simulink model "working_kalman"  (R2025b)
settings: Solver=FixedStepDiscrete  StartTime=0.0  StopTime=+inf  FixedStep=simulink_Ts  RelTol=1e-3  EnableMultiTasking=on
InitFcn:
  | InitSensorFusion
values from neighbouring files (symbols this model uses):
  acc_calib_matrix = [0.9990,0.0039,0.0028;4.2507e-04,0.9990,-0.0085;0.0015,0.0090,0.9997]    [InitSensorFusion.m]
  avg_order = 2    [InitSensorFusion.m]
  calibration_time = 10    [InitSensorFusion.m]
  d = 0.15*sqrt(2)/2    [InitSensorFusion.m]
  friction_offset = 0.0001    [InitSensorFusion.m]
  friction_slope = 20e-6    (= 2e-05)    [InitSensorFusion.m]
  g = 9.81    [InitSensorFusion.m]
  ground_true_g = 9.81275    [InitSensorFusion.m]
  Ic0 = Is0 + Iw0 - Iwg    [InitSensorFusion.m]
  ICM42_gyr_offset = [-0.1319, -0.6878, 0.1737]    [InitSensorFusion.m]
  ICM42_params = SUPER_PARAMS    [InitSensorFusion.m]
  init_acc_bias = [-0.0076;0.0233;0.0477]    [InitSensorFusion.m]
  init_P = P_initial    [InitSensorFusion.m]
  init_rot_quat = [0 0 0 1]'    [InitSensorFusion.m]
  Iwg = 315e-6    (= 0.000315)    [InitSensorFusion.m]
  kalman_Ts = 0.01    [InitSensorFusion.m]
  KV = 330    [InitSensorFusion.m]
  mc = mw + ms    (= 0.75)    [InitSensorFusion.m]
  sensor_Ts = 0.01    [InitSensorFusion.m]
  simulink_Ts = 0.01    [InitSensorFusion.m]
  stateInit = StateEnum.Initialization    [InitSensorFusion.m]
undefined symbols (not defined in the file or in its folder): acc_init_bias, init_time, StateEnum
libraries: mbedblockslib x25, simulink x12, nucleoutilitieslib x10, stmnucleof7lib x7, canmsglib x6, simulink_extras x2, visionstatistics x2
(part 1 of 2)
settings Model: SimulationMode=external  ExtModeTrigDuration=10  Creator=dozav  LastModifiedBy=dozav
settings SolverCC: AutoInsertRateTranBlk=on
settings DataIOCC: SaveOutput=off  DSMLogging=off  ReturnWorkspaceOutputs=off  LoggingFileName=loggedData.mat
settings OptimizationCC: EnhancedBackFolding=on  PassReuseOutputArgsAs=Individual arguments  ZeroExternalMemoryAtStartup=off  ZeroInternalMemoryAtStartup=off  MaxStackSize=64  OptimizeBlockOrder=speed  DifferentSizesBufferReuse=on  OptimizationCustomize=off  EfficientTunableParamExpr=on
settings DebuggingCC: ParameterTunabilityLossMsg=error
settings HardwareCC: ProdBitPerPointer=32.0  ProdBitPerSizeT=32.0  ProdBitPerPtrDiffT=32.0  ProdLargestAtomicInteger=Long  ProdLargestAtomicFloat=Double  ProdWordSize=32.0  ProdLongLongMode=on  ProdHWDeviceType=ARM Compatible->ARM Cortex-M
settings ModelReferenceCC: UpdateModelReferenceTargets=Force
settings SFSimCC: MATLABDynamicMemAlloc=off
settings RTWCC: SystemTargetFile=ert.tlc  HardwareBoard=STM32 Nucleo F767ZI  TemplateMakefile=ert_default_tmf  Toolchain=GNU Tools for ARM Embedded Processors  Description=Embedded Coder
settings CodeAppCC: ForceParamTrailComments=on  IgnoreCustomStorageClasses=off  OperatorAnnotations=on  SimulinkDataObjDesc=on  SFDataObjDesc=on  InsertBlockDesc=on
settings ERTTargetCC: ExtModeTransport=3.0  ExtModeStaticAlloc=on  ExtModeStaticAllocSize=2000.0  ExtModeMexFile=ext_xcp  ExtModeIntrfLevel=Level2 - Open  InlinedParameterPlacement=Hierarchical  TargetLangStandard=C99 (ISO)

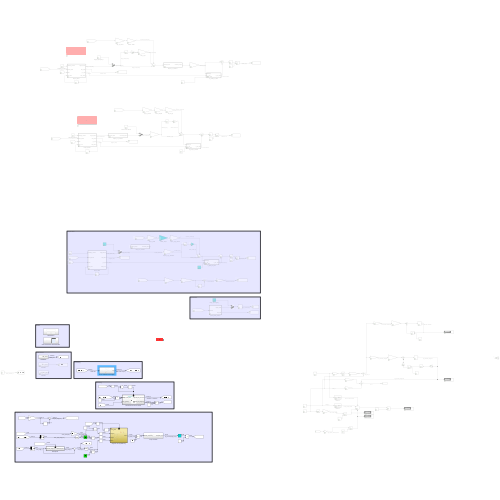
[thumbnail: Simulink's stored preview of the top-level diagram]
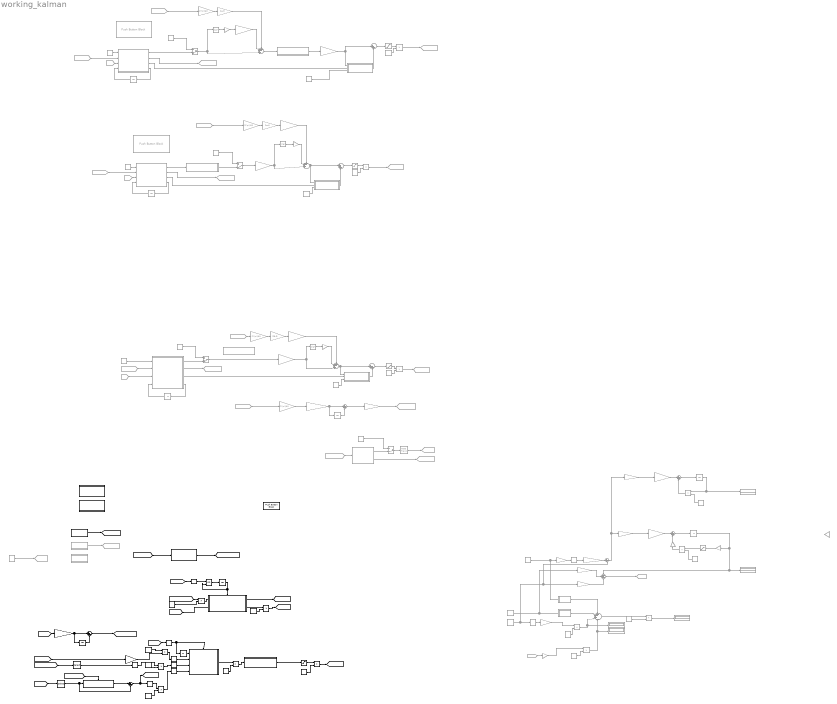
== system working_kalman ==
  note: Regulation
  note: Torque stairs
  note: Speed stairs
  note: Utilities
  note: Estimating
  note: Processing
  note: Measurement
  CAN communication with B-G431-ESC1 : Subsystem
  Constant{1,8..9,16,21} (5 alike) : Constant
  Constant{2,4,6,10..12,19..20} (8 alike) : Constant  Commented=on
  Constant13 : Constant  Commented=on  Value=0
  Constant14 : Constant  Commented=on  Value=0
  Constant15 : Constant  Commented=on  Value=0
  Constant17 : Constant  Value=-1
  Constant18 : Constant  Value=-1
  Constant3 : Constant  Commented=on  Value=5
  Constant5 : Constant  Commented=on  Value=5
  Constant7 : Constant  Commented=on  Value=5
  Degrees to Radians : simulink_extras/Transformations/Degrees to Radians
  Degrees to Radians1 : simulink_extras/Transformations/Degrees to Radians
  Display{,1..4} (5 alike) : Display  Commented=on
  Friction2 : Subsystem  Commented=on
  Friction3 : Subsystem  Commented=on
  From : From  Commented=on  GotoTag=seconds_counter  TagVisibility=global
  From{10..11,13..14,16..17,19} (7 alike) : From  Commented=on  GotoTag=wheel_speed  TagVisibility=global
  From12 : From  Commented=on  GotoTag=state  TagVisibility=global
  From15 : From  Commented=on  GotoTag=state  TagVisibility=global
  From18 : From  Commented=on  GotoTag=state  TagVisibility=global
  From29 : From  Commented=on  GotoTag=v
  Gain : Gain  Gain=1/kalman_Ts
  Gain1 : Gain  Gain=2*pi/60
  Gain10 : Gain  Commented=on  Gain=(2*pi*KV)/60
  Gain11 : Gain  Commented=on  Gain=0.2
  Gain12 : Gain  Commented=on  Gain=11
  Gain13 : Gain  Commented=on  Gain=Ic0
  Gain14 : Gain  Commented=on  Gain=Ic0
  Gain15 : Gain  Commented=on  Gain=-36
  Gain16 : Gain  Commented=on  Gain=-0.02
  Gain17 : Gain  Commented=on  Gain=1/Ic0
  Gain18 : Gain  Commented=on  Gain=Ic0
  Gain19 : Gain  Commented=on  Gain=mc*g*d
  Gain2 : Gain  Commented=on  Gain=simulink_Ts
  Gain20 : Gain  Commented=on  Gain=0.15
  Gain22 : Gain  Commented=on  Gain=-36
  Gain24 : Gain  Commented=on  Gain=simulink_Ts
  Gain3 : Gain  Commented=on  Gain=1/(simulink_Ts*2)
  Gain4 : Gain  Commented=on  Gain=36
  Gain5 : Gain  Commented=on  Gain=Iwg
  Gain6 : Gain  Commented=on  Gain=(2*pi)/60
  Gain7 : Gain  Commented=on  Gain=0.2
  Gain8 : Gain  Commented=on  Gain=(2*pi*KV)/60
  Gain9 : Gain  Commented=on  Gain=0.2
  Goto10 : Goto  Commented=on  GotoTag=applied_torque
  Goto{7,11..12,14} (4 alike) : Goto  Commented=on  GotoTag=program_stop  TagVisibility=global
  Goto13 : Goto  Commented=on  GotoTag=ramp_torque  TagVisibility=global
  Goto15 : Goto  Commented=on  GotoTag=ramp_torque  TagVisibility=global
  Goto16 : Goto  Commented=on  GotoTag=check_timer
  Goto17 : Goto  Commented=on  GotoTag=v
  Goto5 : Goto  Commented=on  GotoTag=MPU_AccGyr
  Goto6 : Goto  Commented=on  GotoTag=ramp_speed  TagVisibility=global
  Goto9 : Goto  Commented=on  GotoTag=ramp_torque  TagVisibility=global
  ICM20948 : Subsystem  Commented=on
  ICM42688-P : Subsystem
  Iq_peak_for_start : MATLAB Function  Commented=on  TreatAsAtomicUnit=on
  Iq_peak_for_start1 : MATLAB Function  Commented=on  TreatAsAtomicUnit=on
  Iq_peak_for_start2 : MATLAB Function  Commented=on  TreatAsAtomicUnit=on
  Kalman Sensor Fusion for ICM42 : Subsystem
  MPU6050 : Subsystem  Commented=on
  Manual Switch{,1..3} (4 alike) : ManualSwitch  Commented=on  CurrentSetting=0
  New Setpoint : Subsystem
  Nm_to_Iq1 : Gain  Commented=on  Gain=1/((2*pi*KV)/60)
  Nm_to_Iq2 : Gain  Commented=on  Gain=(2*pi*KV)/60
  OR : Logic  Operator=OR  IconShape=distinctive  AllPortsSameDT=off  OutDataTypeStr=boolean
  Product{,4..5,10..12,14} (7 alike) : Product
  Product{1..3,6..9,13} (8 alike) : Product  Commented=on
  Push Button : PushButtonBlock  ButtonText=Start/Stop  IconOnColor=[0.0, 0.39215686274509803, 0.0]  IconOffColor=[0.0, 1.0, 0.0]  OffValue=0.000000
  Push Button1 : PushButtonBlock  Commented=on  ButtonText=Start/Stop  IconOnColor=[0.0, 0.39215686274509803, 0.0]  IconOffColor=[0.0, 1.0, 0.0]  OffValue=0.000000
  Push Button2 : PushButtonBlock  Commented=on  ButtonText=Start/Stop  IconOnColor=[0.0, 0.39215686274509803, 0.0]  IconOffColor=[0.0, 1.0, 0.0]  OffValue=0.000000
  Rate Transition{,1..3} (4 alike) : RateTransition  OutPortSampleTime=simulink_Ts
  Rate Transition4 : RateTransition  Commented=on  OutPortSampleTime=simulink_Ts
  Rate Transition5 : RateTransition  OutPortSampleTime=kalman_Ts
  Regulation for Edge Balancing : Subsystem
  Saturation : Saturate  UpperLimit=4  LowerLimit=-4
  Saturation1 : Saturate  Commented=on  UpperLimit=4.5  LowerLimit=-4.5
  Saturation2 : Saturate  Commented=on  UpperLimit=1.8  LowerLimit=-1.8
  Saturation3 : Saturate  Commented=on  UpperLimit=1.8  LowerLimit=-1.8
  Saturation4 : Saturate  Commented=on
  Selector : Selector  InputPortWidth=3  IndexOptions=Index vector (dialog)  Indices=[3]  OutputSizes=1
  Selector1 : Selector  InputPortWidth=3  IndexOptions=Index vector (dialog)  Indices=[3]  OutputSizes=1
  Sensor Calibration and Averaging : Subsystem
  Sign : Signum  Commented=on
  Sign1 : Signum  Commented=on
  Sign2 : Signum  Commented=on
  Sin3 : Trigonometry  Commented=on
  State Machine : Subsystem
  Sum : Sum  Inputs=|+-
  Sum1 : Sum  Inputs=|+-
  Sum10 : Sum  Commented=on  Inputs=---
  Sum11 : Sum  Commented=on  Inputs=|+-
  Sum12 : Sum  Commented=on  Inputs=+|-|+|-
  Sum{4,6,8..9,13} (5 alike) : Sum  Commented=on  Inputs=|++
  Sum2 : Sum  Commented=on  Inputs=|+-
  Sum3 : Sum  Commented=on  Inputs=+++|
  Sum5 : Sum  Commented=on  Inputs=+++|
  Sum7 : Sum  Commented=on  Inputs=+++|
  Tanh1 : Trigonometry  Commented=on  Operator=tanh
  Torque Correction : Subsystem
  Unit Delay : UnitDelay  SampleTime=-1  HasFrameUpgradeWarning=on
  Unit Delay{1..2,6..8} (5 alike) : UnitDelay  Commented=on  SampleTime=simulink_Ts  HasFrameUpgradeWarning=on
  Unit Delay3 : UnitDelay  InitialCondition=zeros(1,3)  SampleTime=kalman_Ts  HasFrameUpgradeWarning=on
  Unit Delay4 : UnitDelay  SampleTime=simulink_Ts  HasFrameUpgradeWarning=on
  Unit Delay5 : UnitDelay  Commented=on  SampleTime=simulink_Ts*2  HasFrameUpgradeWarning=on
  friction_slope : Gain  Commented=on  Gain=2e-5
  friction_slope1 : Gain  Commented=on  Gain=2e-5
  friction_slope2 : Gain  Commented=on  Gain=2e-5
  manual_target_torque [Nm] : Constant  Commented=on  Value=0.01  OutDataTypeStr=single
  rpm_to_rad/s : Gain  Commented=on  Gain=(2*pi)/60
  rpm_to_rad/s1 : Gain  Commented=on  Gain=(2*pi)/60
  rpm_to_rad/s2 : Gain  Commented=on  Gain=(2*pi)/60
  sampling_counter{,1..3} (4 alike) : simulink/Sources/Counter Free-Running  Commented=on  NumBits=32  tsamp=simulink_Ts
  speed_stairs_function : MATLAB Function  Commented=on  TreatAsAtomicUnit=on
  target_speed [rpm] : Constant  Commented=on  Value=1500  OutDataTypeStr=single
  target_torque [Nm]1 : Constant  Commented=on  Value=0.01  OutDataTypeStr=single
  target_torque [Nm]2 : Constant  Commented=on  Value=0.01  OutDataTypeStr=single
  torque_inv_function : MATLAB Function  Commented=on  TreatAsAtomicUnit=on
  torque_inv_function1 : MATLAB Function  Commented=on  TreatAsAtomicUnit=on
  torque_inv_function2 : MATLAB Function  Commented=on  TreatAsAtomicUnit=on
  torque_stairs : MATLAB Function  Commented=on  TreatAsAtomicUnit=on
  torque_stairs1 : MATLAB Function  Commented=on  TreatAsAtomicUnit=on
  torque_stairs2 : MATLAB Function  Commented=on  TreatAsAtomicUnit=on
  torque_to_Iq_corrected : Gain  Commented=on  Gain=(2*pi*KV)/60
  torque_to_Iq_friction : Gain  Commented=on  Gain=(2*pi*KV)/60
  tag scope: ICM42_EA=global, ICM42_rot_q=global, error_angle=global, ramp_torque=global
  wires:
  ICM42688-P/1(ICM_AccGyr) -> [ICM42_AccGyr]  "ICM42_data"
  [ICM42_g] -> Kalman Sensor Fusion for ICM42/2(used_g [m/s^2])
  MPU6050/1(MPU_AccGyr) -> Goto5/1
  [isIdle] -> Rate Transition5/1
  OR/1 -> Unit Delay/1
  [ICM42_AccGyr] -> Sensor Calibration and Averaging/1(In1)  "ICM42_data"
  Sensor Calibration and Averaging/1(avg) -> [ICM42_AccGyr_avg]  "ICM42_data_avg"
  Kalman Sensor Fusion for ICM42/1(Out1) -> [ICM42_rot_q]  "estimated_rot_quaternion"
  Gain/1 -> Sum/1, Unit Delay3/1
  [wheel_speed] -> Gain1/1  "wheel_speed [rpm]"
  Sum/1 -> [ICM42_EA_omega]  "ICM_EA_omega [°/s]"
  Torque Correction/1(corrected_Iq [A]) -> Saturation/1  "reg_corrected_target_Iq [A]"
  [ICM42_EA] -> Gain/1
  [ICM42_EA_omega] -> Selector1/1
  Selector1/1 -> Degrees to Radians/1  "euler_angle_omega [°/s]"
  Unit Delay3/1 -> Sum/2
  Sum1/1 -> [error_angle], Degrees to Radians1/1  "error_angle [°]"
  Product/1 -> [ramp_torque]
  Constant1/1 -> Product/2
  Rate Transition/1 -> Regulation for Edge Balancing/4(theta c)
  Rate Transition1/1 -> Regulation for Edge Balancing/3(omega c)
  [isRunning] -> Rate Transition3/1
  Rate Transition3/1 -> Regulation for Edge Balancing/Enable, Unit Delay4/1
  Unit Delay4/1 -> Regulation for Edge Balancing/1(running_label)
  From/1 -> speed_stairs_function/1(seconds)
  speed_stairs_function/2(stop_start) -> Goto7/1
  speed_stairs_function/1(target_speed) -> Manual Switch/2
  Manual Switch/1 -> Rate Transition4/1
  target_speed [rpm]/1 -> Manual Switch/1
  Rate Transition4/1 -> Goto6/1  "target_speed [rpm]"
  manual_target_torque [Nm]/1 -> Manual Switch1/1
  Gain3/1 -> Sum2/1, Unit Delay5/1
  Unit Delay5/1 -> Sum2/2
  Gain6/1 -> Gain3/1
  Sum2/1 -> Gain5/1  "rot_accel [rad/s^2]"
  Gain5/1 -> Goto10/1  "applied_torque [Nm]"
  From10/1 -> Gain6/1
  torque_stairs/2(stop_start) -> Goto11/1  "program_stop"
  torque_stairs/1(target_torque) -> Manual Switch1/2  "target_torque [Nm]"
  Saturation1/1 -> Product1/1
  Constant2/1 -> Product1/2
  Product1/1 -> Goto9/1  "target_Iq [A]"
  Manual Switch1/1 -> torque_to_Iq_corrected/1  "target_torque [Nm]"
  sampling_counter/1 -> torque_stairs/1(sampling_counter)
  From11/1 -> torque_stairs/2(wheel_speed)
  From12/1 -> torque_stairs/3(state)
  torque_stairs/4(step_done) -> Unit Delay6/1
  Unit Delay6/1 -> torque_stairs/4("step_done ")
  torque_stairs/3(t_in_slot) -> Iq_peak_for_start/2(t_in_slot)  "t_in_slot [s]"
  torque_to_Iq_corrected/1 -> Sum3/3, Sign/1  "desired_Iq [A]"
  Constant3/1 -> Iq_peak_for_start/3(decay_slope)
  Sign/1 -> Gain7/1
  Sum3/1 -> Iq_peak_for_start/1(desired_Iq), Sum4/1
  Iq_peak_for_start/1(Iq_for_start) -> Sum4/2  "Iq_peak_ampl [A]"
  Sum4/1 -> Saturation1/1
  From13/1 -> rpm_to_rad/s/1
  Gain7/1 -> Sum3/2  "static_friction [A]"
  rpm_to_rad/s/1 -> friction_slope/1
  friction_slope/1 -> torque_to_Iq_friction/1
  torque_to_Iq_friction/1 -> Sum3/1  "dynamic_friction [A]"
  friction_slope1/1 -> Sum5/1  "dynamic_torque [Nm]"
  Product2/1 -> Goto13/1  "target_Iq [A]"
  Sum5/1 -> torque_inv_function1/1(desired_torque)
  torque_stairs1/2(stop_start) -> Goto12/1  "program_stop"
  target_torque [Nm]1/1 -> Manual Switch2/1
  Sign1/1 -> Gain9/1
  torque_stairs1/1(target_torque) -> Manual Switch2/2  "target_torque [Nm]"
  From14/1 -> torque_stairs1/2(wheel_speed)
  Manual Switch2/1 -> Sum5/3, Sign1/1  "target_torque [Nm]"
  Saturation2/1 -> Product2/1
  Constant4/1 -> Product2/2
  From15/1 -> torque_stairs1/3(state)
  Constant5/1 -> Iq_peak_for_start1/3(decay_slope)
  Unit Delay7/1 -> torque_stairs1/4("step_done ")
  rpm_to_rad/s1/1 -> friction_slope1/1
  Sum6/1 -> Saturation2/1
  torque_stairs1/3(t_in_slot) -> Iq_peak_for_start1/2(t_in_slot)  "t_in_slot [s]"
  Iq_peak_for_start1/1(Iq_for_start) -> Sum6/2  "Iq_peak_ampl [A]"
  sampling_counter1/1 -> torque_stairs1/1(sampling_counter)
  From16/1 -> rpm_to_rad/s1/1
  Gain9/1 -> Nm_to_Iq1/1  "static_friction [A]"
  torque_stairs1/4(step_done) -> Unit Delay7/1
  Nm_to_Iq1/1 -> Sum5/2  "static_torque [Nm]"
  Gain8/1 -> Sum6/1, Iq_peak_for_start1/1(desired_Iq)  "desired_Iq [A]"
  torque_inv_function1/1(corrected_torque) -> Gain8/1
  friction_slope2/1 -> Nm_to_Iq2/1
  Gain10/1 -> Sign2/1, Sum7/3  "desired_Iq [A]"
  Unit Delay8/1 -> torque_stairs2/4("step_done ")
  Sum7/1 -> Iq_peak_for_start2/1(desired_Iq), Sum8/1
  torque_stairs2/2(stop_start) -> Goto14/1  "program_stop"
  torque_stairs2/3(t_in_slot) -> Iq_peak_for_start2/2(t_in_slot)  "t_in_slot [s]"
  From18/1 -> torque_stairs2/3(state)
  Constant7/1 -> Iq_peak_for_start2/3(decay_slope)
  Gain11/1 -> Sum7/2  "static_friction [A]"
  From17/1 -> torque_stairs2/2(wheel_speed)
  Constant6/1 -> Product3/2
  target_torque [Nm]2/1 -> Manual Switch3/1
  rpm_to_rad/s2/1 -> friction_slope2/1
  Sum8/1 -> Saturation3/1
  From19/1 -> rpm_to_rad/s2/1
  torque_stairs2/4(step_done) -> Unit Delay8/1
  Nm_to_Iq2/1 -> Sum7/1  "dynamic_friction [A]"
  sampling_counter2/1 -> torque_stairs2/1(sampling_counter)
  Product3/1 -> Goto15/1  "target_Iq [A]"
  Sign2/1 -> Gain11/1
  Saturation3/1 -> Product3/1
  torque_inv_function2/1(corrected_torque) -> Manual Switch3/2
  torque_stairs2/1(target_torque) -> torque_inv_function2/1(desired_torque)  "target_torque [Nm]"
  Manual Switch3/1 -> Gain10/1  "target_torque [Nm]"
  Iq_peak_for_start2/1(Iq_for_start) -> Sum8/2  "Iq_peak_ampl [A]"
  Saturation/1 -> Product/1
  sampling_counter3/1 -> Goto16/1  "timer_simulink_Ts"
  Constant8/1 -> Product4/2
  Regulation for Edge Balancing/1(torque) -> Product4/1  "reg_target_torque [Nm]"
  Product4/1 -> Torque Correction/1(desired_torque [Nm])
  Constant9/1 -> Product5/2
  Kalman Sensor Fusion for ICM42/2(EA) -> Product5/1  "estimated_euler_angles [°]"
  Product5/1 -> [ICM42_EA]
  Rate Transition2/1 -> Regulation for Edge Balancing/2(omega w)
  Constant16/1 -> Product10/1
  Gain1/1 -> Product10/2  "wheel_speed [rad/s]"
  Product10/1 -> Rate Transition2/1
  Sum9/1 -> Unit Delay1/1
  Sin3/1 -> Gain19/1
  Product7/1 -> Display/1
  Gain20/1 -> Tanh1/1
  Gain2/1 -> Sum9/1
  Sum10/1 -> Goto17/1  "reg_v"
  Gain16/1 -> Sum11/1
  Tanh1/1 -> Gain16/1
  Gain12/1 -> Sum10/2
  Gain18/1 -> Product8/1  "reg_torque_fictional_action"
  Constant19/1 -> Product6/2
  Sum12/1 -> Product7/1
  Constant12/1 -> Product9/2
  Constant11/1 -> Product7/2
  Gain19/1 -> Product9/1  "reg_torque_gravity"
  Constant15/1 -> Gain12/1, Friction3/1(rad/s)  "omega_c"
  Unit Delay1/1 -> Display4/1, Sum10/1, Gain13/1  "reg_discrete_integrator"
  Constant13/1 -> Friction2/1(rad/s), Gain20/1
  Friction3/1(friction) -> Sum12/2  "torque_cubli_friction"
  Constant14/1 -> Gain4/1, Sum11/2, Sin3/1  "theta_c"
  From29/1 -> Gain18/1
  Gain4/1 -> Sum10/3
  Product6/1 -> Gain17/1
  Product9/1 -> Sum12/3, Display1/1
  Product8/1 -> Display2/1, Sum12/4
  Constant10/1 -> Product8/2
  Friction2/1(friction) -> Sum12/1  "torque_wheel_friction"
  Constant17/1 -> Product11/2
  Degrees to Radians1/1 -> Product11/1  "error_euler_angle [rad]"
  Product11/1 -> Rate Transition/1
  Constant18/1 -> Product12/2
  Degrees to Radians/1 -> Product12/1  "euler_angle_omega [rad/s]"
  Product12/1 -> Rate Transition1/1
  Saturation4/1 -> Product6/1
  Sum11/1 -> Gain22/1, Gain15/1  "reg_thc_err"
  Gain15/1 -> Gain2/1  "reg_discrete_integrator"
  Gain13/1 -> Saturation4/1
  Gain17/1 -> Sum9/2
  Constant20/1 -> Product13/2
  Gain22/1 -> Gain24/1  "reg_discrete_integrator"
  Gain24/1 -> Sum13/1
  Sum13/1 -> Unit Delay2/1
  Unit Delay2/1 -> Display3/1, Product13/1  "reg_discrete_integrator"
  Product13/1 -> Sum13/2
  Constant21/1 -> Product14/2
  [ICM42_AccGyr_avg] -> Product14/1
  Product14/1 -> Kalman Sensor Fusion for ICM42/1(meased_data_6axis)
  Unit Delay/1 -> OR/2, Kalman Sensor Fusion for ICM42/Enable
  Rate Transition5/1 -> OR/1
  [isSettingSetpoint] -> New Setpoint/Enable
  [ICM42_EA] -> Selector/1
  Selector/1 -> New Setpoint/1(measured_angle [°]), Sum1/2  "euler_angle [°]"
  New Setpoint/1(setpoint_angle [°]) -> Sum1/1  "target_angle [°]"

== system working_kalman/CAN communication with B-G431-ESC1 ==
  Receive CAN Messages : Subsystem
  Send CAN Messages : Subsystem

== system working_kalman/Friction2 ==
  rad/s : Inport
  Gain : Gain  Gain=300
  Gain1 : Gain  Gain=friction_offset
  Gain2 : Gain  Gain=friction_slope
  Gain4 : Gain  Gain=1/(2*pi*60)
  Sum : Sum  Inputs=|++
  Tanh : Trigonometry  Operator=tanh
  friction : Outport
  wires:
  rad/s/1 -> Gain4/1
  Gain4/1 -> Gain2/1, Gain/1  "rpm"
  Gain1/1 -> Sum/1
  Tanh/1 -> Gain1/1
  Gain2/1 -> Sum/2
  Gain/1 -> Tanh/1
  Sum/1 -> friction/1

== system working_kalman/Friction3 ==
  rad/s : Inport
  Gain : Gain  Gain=300
  Gain1 : Gain  Gain=friction_offset
  Gain2 : Gain  Gain=friction_slope
  Gain4 : Gain  Gain=1/(2*pi*60)
  Sum : Sum  Inputs=|++
  Tanh : Trigonometry  Operator=tanh
  friction : Outport
  wires:
  rad/s/1 -> Gain4/1
  Gain4/1 -> Gain2/1, Gain/1  "rpm"
  Gain1/1 -> Sum/1
  Tanh/1 -> Gain1/1
  Gain2/1 -> Sum/2
  Gain/1 -> Tanh/1
  Sum/1 -> friction/1

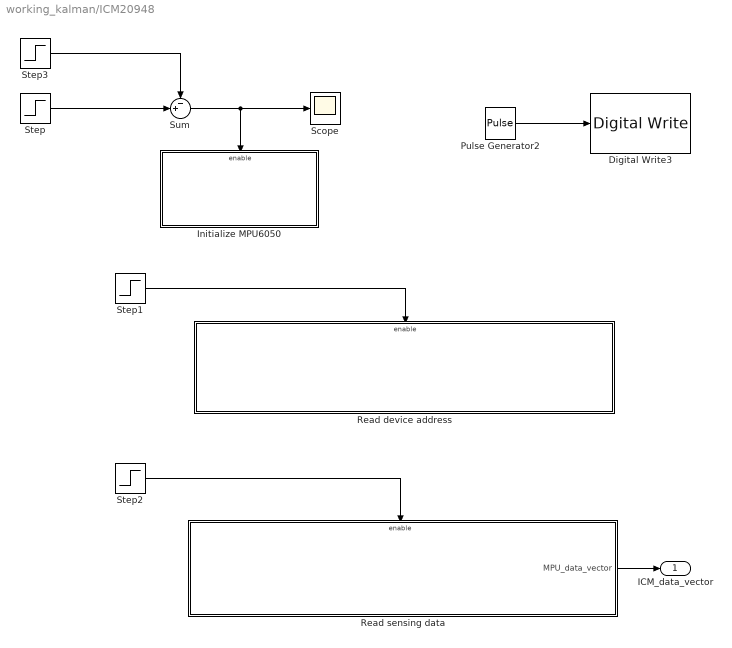
== system working_kalman/ICM20948 ==
  Digital Write3 : mbedblockslib/Digital Write  Pin=LED3  Direction=output
      settings: LibrarySourceBlock=stmnucleorootlib/Common/Digital Write
  Initialize MPU6050 : Subsystem
  Pulse Generator2 : DiscretePulseGenerator  PulseType=Time based  PulseWidth=50
  Read device address : Subsystem
  Read sensing data : Subsystem
  Scope : Scope
      settings: DataLoggingVariableName=ScopeData5
  Step : Step
  Step1 : Step  Time=2
  Step2 : Step  Time=2
  Step3 : Step  Time=1.5
  Sum : Sum  Inputs=-+|
  ICM_data_vector : Outport
  wires:
  Step2/1 -> Read sensing data/Enable
  Read sensing data/1(MPU_data_vector) -> ICM_data_vector/1
  Sum/1 -> Scope/1, Initialize MPU6050/Enable
  Step/1 -> Sum/2
  Step1/1 -> Read device address/Enable
  Step3/1 -> Sum/1
  Pulse Generator2/1 -> Digital Write3/1

== system working_kalman/ICM42688-P ==
  Measurement : Subsystem
  OR : Logic  Operator=OR  IconShape=distinctive  AllPortsSameDT=off  OutDataTypeStr=boolean
  Range and sensitivity : Subsystem  Priority=1
  Selector : Selector  InputPortWidth=7  IndexOptions=Starting index (dialog)  Indices=[2]  OutputSizes=6
  Step1 : Step  Time=init_time - 3
  Step3 : Step  Time=init_time - 4
  Unit Delay : UnitDelay  SampleTime=-1  HasFrameUpgradeWarning=on
  Waking up : Subsystem  Priority=2
  ICM_AccGyr : Outport
  wires:
  Step1/1 -> Waking up/Trigger
  Step3/1 -> Range and sensitivity/Trigger
  OR/1 -> Unit Delay/1
  Unit Delay/1 -> OR/2, Measurement/Enable
  Measurement/1(ICM_data_vector) -> Selector/1
  [isCalibrating] -> OR/1
  Selector/1 -> ICM_AccGyr/1

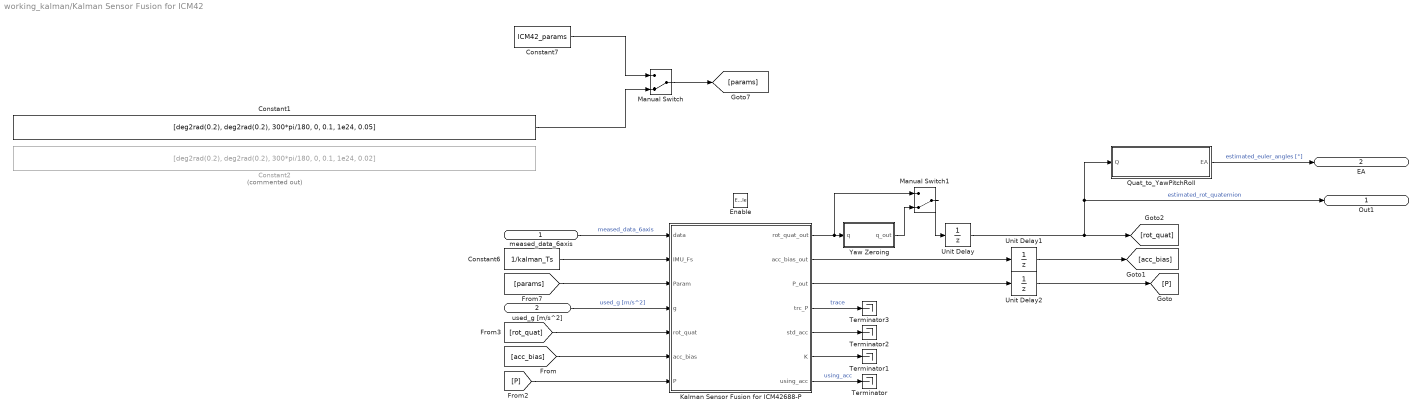
== system working_kalman/Kalman Sensor Fusion for ICM42 ==
  meased_data_6axis : Inport
  used_g [m/s^2] : Inport  Port=2
  Enable : EnablePort
  Constant1 : Constant  Value=[deg2rad(0.2), deg2rad(0.2), 300*pi/180, 0, 0.1, 1e24, 0.05]  SampleTime=-1
  Constant2 : Constant  Commented=on  Value=[deg2rad(0.2), deg2rad(0.2), 300*pi/180, 0, 0.1, 1e24, 0.02]  SampleTime=-1
  Constant6 : Constant  Value=1/kalman_Ts  SampleTime=kalman_Ts
  Constant7 : Constant  Value=ICM42_params  SampleTime=-1
  Kalman Sensor Fusion for ICM42688-P : MATLAB Function  TreatAsAtomicUnit=on  SystemSampleTime=kalman_Ts
  Manual Switch : ManualSwitch  CurrentSetting=0
  Manual Switch1 : ManualSwitch  CurrentSetting=0
  Quat_to_YawPitchRoll : MATLAB Function  TreatAsAtomicUnit=on
  Terminator{,1..3} (4 alike) : Terminator
  Unit Delay : UnitDelay  InitialCondition=init_rot_quat  SampleTime=kalman_Ts  HasFrameUpgradeWarning=on
  Unit Delay1 : UnitDelay  InitialCondition=init_acc_bias  SampleTime=kalman_Ts  HasFrameUpgradeWarning=on
  Unit Delay2 : UnitDelay  InitialCondition=init_P*eye(7)  SampleTime=kalman_Ts  HasFrameUpgradeWarning=on
  Yaw Zeroing : MATLAB Function  TreatAsAtomicUnit=on
  Out1 : Outport
  EA : Outport  Port=2
  wires:
  [acc_bias] -> Kalman Sensor Fusion for ICM42688-P/6(acc_bias)
  [P] -> Kalman Sensor Fusion for ICM42688-P/7(P)
  Unit Delay/1 -> Quat_to_YawPitchRoll/1(Q), Out1/1, [rot_quat]  "estimated_rot_quaternion"
  [rot_quat] -> Kalman Sensor Fusion for ICM42688-P/5(rot_quat)
  Kalman Sensor Fusion for ICM42688-P/2(acc_bias_out) -> Unit Delay1/1
  Kalman Sensor Fusion for ICM42688-P/3(P_out) -> Unit Delay2/1
  [params] -> Kalman Sensor Fusion for ICM42688-P/3(Param)
  Unit Delay1/1 -> [acc_bias]
  Unit Delay2/1 -> [P]
  meased_data_6axis/1 -> Kalman Sensor Fusion for ICM42688-P/1(data)  "meased_data_6axis"
  used_g [m/s^2]/1 -> Kalman Sensor Fusion for ICM42688-P/4(g)  "used_g [m/s^2]"
  Quat_to_YawPitchRoll/1(EA) -> EA/1  "estimated_euler_angles [°]"
  Constant6/1 -> Kalman Sensor Fusion for ICM42688-P/2(IMU_Fs)
  Constant7/1 -> Manual Switch/1
  Constant1/1 -> Manual Switch/2
  Manual Switch/1 -> [params]
  Kalman Sensor Fusion for ICM42688-P/7(using_acc) -> Terminator/1  "using_acc"
  Kalman Sensor Fusion for ICM42688-P/4(trc_P) -> Terminator3/1  "trace"
  Kalman Sensor Fusion for ICM42688-P/5(std_acc) -> Terminator2/1
  Kalman Sensor Fusion for ICM42688-P/6(K) -> Terminator1/1
  Kalman Sensor Fusion for ICM42688-P/1(rot_quat_out) -> Manual Switch1/1, Yaw Zeroing/1(q)
  Manual Switch1/1 -> Unit Delay/1
  Yaw Zeroing/1(q_out) -> Manual Switch1/2

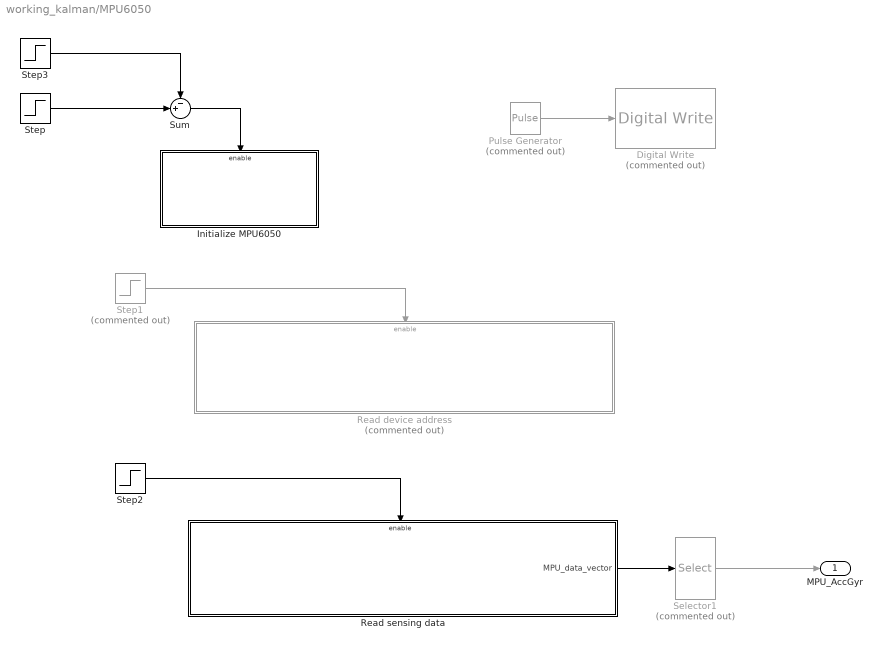
== system working_kalman/MPU6050 ==
  Digital Write : mbedblockslib/Digital Write  Commented=on  Pin=LED1  Direction=output
      settings: LibrarySourceBlock=stmnucleorootlib/Common/Digital Write
  Initialize MPU6050 : Subsystem
  Pulse Generator : DiscretePulseGenerator  Commented=on  PulseType=Time based  Period=0.5  PulseWidth=50
  Read device address : Subsystem  Commented=on
  Read sensing data : Subsystem
  Selector1 : Selector  Commented=on  InputPortWidth=7  IndexOptions=Index vector (dialog)  Indices=[1 2 3 5 6 7]  OutputSizes=6
  Step : Step
  Step1 : Step  Commented=on  Time=2
  Step2 : Step  Time=2
  Step3 : Step  Time=1.5
  Sum : Sum  Inputs=-+|
  MPU_AccGyr : Outport
  wires:
  Step2/1 -> Read sensing data/Enable
  Read sensing data/1(MPU_data_vector) -> Selector1/1
  Sum/1 -> Initialize MPU6050/Enable
  Step/1 -> Sum/2
  Pulse Generator/1 -> Digital Write/1
  Step1/1 -> Read device address/Enable
  Step3/1 -> Sum/1
  Selector1/1 -> MPU_AccGyr/1

== system working_kalman/New Setpoint ==
  measured_angle [°] : Inport
  Enable : EnablePort
  setpoint_angle [°] : Outport  InitialOutput=0
  wires:
  measured_angle [°]/1 -> setpoint_angle [°]/1

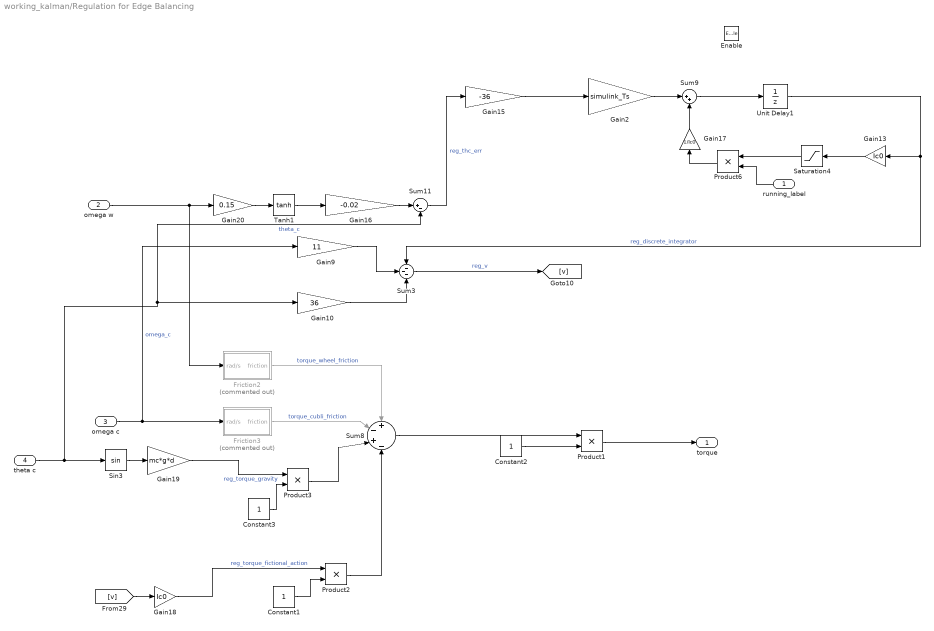
== system working_kalman/Regulation for Edge Balancing ==
  running_label : Inport
  omega w : Inport  Port=2
  omega c : Inport  Port=3
  theta c : Inport  Port=4
  Enable : EnablePort
  Constant1 : Constant
  Constant2 : Constant
  Constant3 : Constant
  Friction2 : Subsystem  Commented=on
  Friction3 : Subsystem  Commented=on
  Gain10 : Gain  Gain=36
  Gain13 : Gain  Gain=Ic0
  Gain15 : Gain  Gain=-36
  Gain16 : Gain  Gain=-0.02
  Gain17 : Gain  Gain=1/Ic0
  Gain18 : Gain  Gain=Ic0
  Gain19 : Gain  Gain=mc*g*d
  Gain2 : Gain  Gain=simulink_Ts
  Gain20 : Gain  Gain=0.15
  Gain9 : Gain  Gain=11
  Product{1..3,6} (4 alike) : Product
  Saturation4 : Saturate
  Sin3 : Trigonometry
  Sum11 : Sum  Inputs=|+-
  Sum3 : Sum  Inputs=---
  Sum8 : Sum  Inputs=+|-|+|-
  Sum9 : Sum  Inputs=|++
  Tanh1 : Trigonometry  Operator=tanh
  Unit Delay1 : UnitDelay  SampleTime=simulink_Ts  HasFrameUpgradeWarning=on
  torque : Outport
  wires:
  omega c/1 -> Gain9/1, Friction3/1(rad/s)  "omega_c"
  Sin3/1 -> Gain19/1
  Sum3/1 -> [v]  "reg_v"
  Friction2/1(friction) -> Sum8/1  "torque_wheel_friction"
  Product1/1 -> torque/1
  Gain16/1 -> Sum11/1
  Gain10/1 -> Sum3/3
  Constant2/1 -> Product1/2
  Tanh1/1 -> Gain16/1
  Friction3/1(friction) -> Sum8/2  "torque_cubli_friction"
  Gain20/1 -> Tanh1/1
  [v] -> Gain18/1
  omega w/1 -> Friction2/1(rad/s), Gain20/1
  Sum8/1 -> Product1/1
  theta c/1 -> Gain10/1, Sum11/2, Sin3/1  "theta_c"
  Gain9/1 -> Sum3/2
  Constant1/1 -> Product2/2
  Gain18/1 -> Product2/1  "reg_torque_fictional_action"
  Product2/1 -> Sum8/4
  Constant3/1 -> Product3/2
  Gain19/1 -> Product3/1  "reg_torque_gravity"
  Product3/1 -> Sum8/3
  Gain15/1 -> Gain2/1
  Gain13/1 -> Saturation4/1
  Saturation4/1 -> Product6/1
  Unit Delay1/1 -> Sum3/1, Gain13/1  "reg_discrete_integrator"
  Gain2/1 -> Sum9/1
  Sum9/1 -> Unit Delay1/1
  Product6/1 -> Gain17/1
  Gain17/1 -> Sum9/2
  running_label/1 -> Product6/2
  Sum11/1 -> Gain15/1  "reg_thc_err"

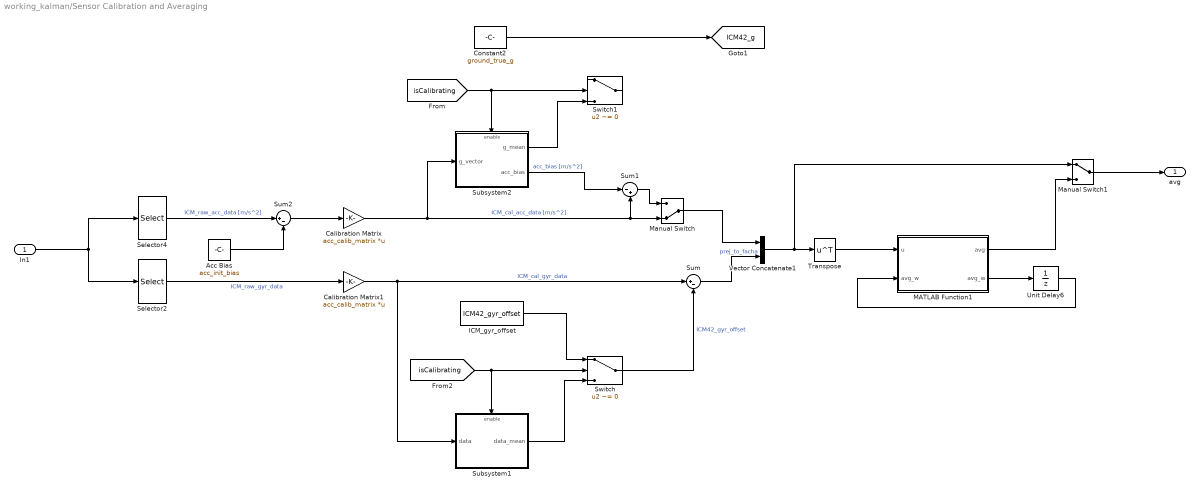
== system working_kalman/Sensor Calibration and Averaging ==
  In1 : Inport
  Acc Bias : Constant  Value=acc_init_bias  SampleTime=simulink_Ts
  Calibration Matrix : Gain  Gain=acc_calib_matrix  Multiplication=Matrix(K*u)
  Calibration Matrix1 : Gain  Gain=acc_calib_matrix  Multiplication=Matrix(K*u)
  Constant2 : Constant  Value=ground_true_g  SampleTime=kalman_Ts
  ICM_gyr_offset : Constant  Value=ICM42_gyr_offset  SampleTime=-1
  MATLAB Function1 : MATLAB Function  TreatAsAtomicUnit=on
  Manual Switch : ManualSwitch  CurrentSetting=0
  Manual Switch1 : ManualSwitch
  Selector2 : Selector  InputPortWidth=6  IndexOptions=Starting index (dialog)  Indices=[4]  OutputSizes=3
  Selector4 : Selector  InputPortWidth=6  IndexOptions=Starting index (dialog)  Indices=[1]  OutputSizes=3
  Subsystem1 : Subsystem
  Subsystem2 : Subsystem
  Sum : Sum  Inputs=|+-
  Sum1 : Sum  Inputs=|-+
  Sum2 : Sum  Inputs=|+-
  Switch : Switch  Criteria=u2 ~= 0  Threshold=111  SaturateOnIntegerOverflow=off  InputSameDT=off
  Switch1 : Switch  Criteria=u2 ~= 0  SaturateOnIntegerOverflow=off  InputSameDT=off
  Transpose : Math  Operator=transpose
  Unit Delay6 : UnitDelay  InitialCondition=zeros(avg_order, 6)  SampleTime=-1  HasFrameUpgradeWarning=on
  Vector Concatenate1 : Concatenate
  avg : Outport
  tag scope: ICM42_g=global
  wires:
  Subsystem1/1(data_mean) -> Switch/3
  In1/1 -> Selector2/1, Selector4/1
  MATLAB Function1/2(avg_w) -> Unit Delay6/1
  Vector Concatenate1/1 -> Manual Switch1/1, Transpose/1
  Selector2/1 -> Calibration Matrix1/1  "ICM_raw_gyr_data"
  [isCalibrating] -> Subsystem2/Enable, Switch1/2
  Subsystem2/1(g_mean) -> Switch1/3
  Unit Delay6/1 -> MATLAB Function1/2("avg_w ")
  ICM_gyr_offset/1 -> Switch/1
  [isCalibrating] -> Switch/2, Subsystem1/Enable
  Switch/1 -> Sum/2  "ICM42_gyr_offset"
  Sum/1 -> Vector Concatenate1/2  "prej_to_facha"
  Transpose/1 -> MATLAB Function1/1(u)
  Subsystem2/2(acc_bias) -> Sum1/1  "acc_bias [m/s^2]"
  Manual Switch/1 -> Vector Concatenate1/1
  Sum1/1 -> Manual Switch/1
  Calibration Matrix/1 -> Sum1/2, Manual Switch/2, Subsystem2/1(g_vector)  "ICM_cal_acc_data [m/s^2]"
  Selector4/1 -> Sum2/1  "ICM_raw_acc_data [m/s^2]"
  Sum2/1 -> Calibration Matrix/1
  Acc Bias/1 -> Sum2/2
  Constant2/1 -> [ICM42_g]
  Calibration Matrix1/1 -> Sum/1, Subsystem1/1(data)  "ICM_cal_gyr_data"
  MATLAB Function1/1(avg) -> Manual Switch1/2
  Manual Switch1/1 -> avg/1

== system working_kalman/State Machine ==
  State Recognition : Subsystem
  State Signalizition : Subsystem
  State Updates : Subsystem

== system working_kalman/Torque Correction ==
  desired_torque [Nm] : Inport
  Gain12 : Gain  Gain=(2*pi*KV)/60
  Gain13 : Gain  Gain=0.2
  Sign3 : Signum
  Sum9 : Sum  Inputs=+++|
  friction_slope3 : Gain  Gain=2e-5
  friction_torque_to_Iq1 : Gain  Gain=(2*pi*KV)/60
  rpm_to_rad/s3 : Gain  Gain=(2*pi)/60
  torque_inv_function3 : MATLAB Function  TreatAsAtomicUnit=on
  corrected_Iq [A] : Outport
  wires:
  Gain13/1 -> Sum9/2  "offset_for_dynamic_friction [A]"
  rpm_to_rad/s3/1 -> friction_slope3/1
  torque_inv_function3/1(corrected_torque) -> Gain12/1  "corrected_torque [Nm]"
  [wheel_speed] -> rpm_to_rad/s3/1
  Gain12/1 -> Sum9/3, Sign3/1  "desired_Iq [A]"
  Sign3/1 -> Gain13/1
  friction_torque_to_Iq1/1 -> Sum9/1  "dynamic_friction [A]"
  friction_slope3/1 -> friction_torque_to_Iq1/1
  desired_torque [Nm]/1 -> torque_inv_function3/1(desired_torque)  "desired_torque [Nm]"
  Sum9/1 -> corrected_Iq [A]/1  "corrected_Iq [A]"

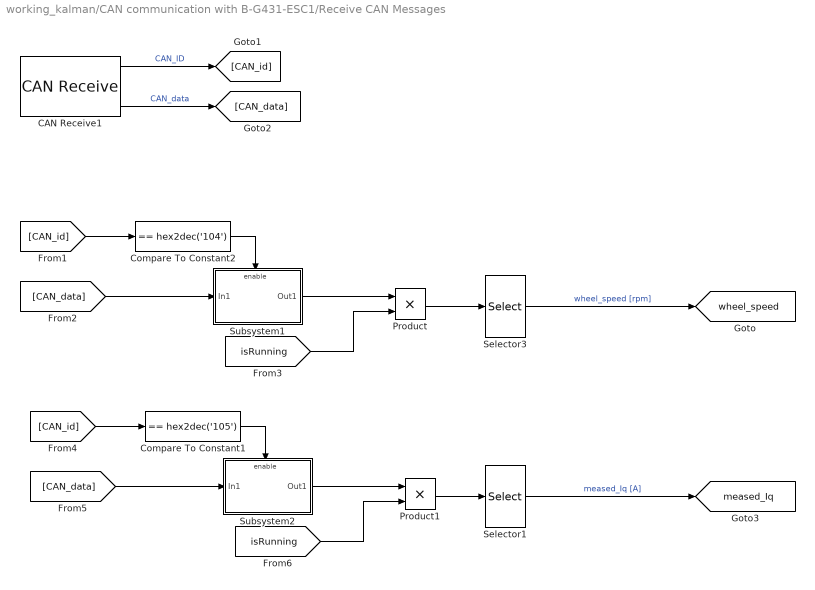
== system working_kalman/CAN communication with B-G431-ESC1/Receive CAN Messages ==
  CAN Receive1 : stmnucleof7lib/CAN Receive  CANModule=1  OutputType=Unpacked  ReadSource=FIFO 0  SampleTime=simulink_Ts  OutputIdType=off  RemoteFrame=off  OutputStatus=off
  Compare To Constant1 : simulink/Logic and Bit Operations/Compare To Constant  relop===  const=hex2dec('105')  OutDataTypeStr=boolean
  Compare To Constant2 : simulink/Logic and Bit Operations/Compare To Constant  relop===  const=hex2dec('104')  OutDataTypeStr=boolean
  Product : Product
  Product1 : Product
  Selector1 : Selector  InputPortWidth=2  IndexOptions=Starting index (dialog)  Indices=[1]  OutputSizes=1
  Selector3 : Selector  InputPortWidth=2  IndexOptions=Starting index (dialog)  Indices=[1]  OutputSizes=1
  Subsystem1 : Subsystem
  Subsystem2 : Subsystem
  tag scope: meased_Iq=global, wheel_speed=global
  wires:
  CAN Receive1/3 -> [CAN_data]  "CAN_data"
  Compare To Constant2/1 -> Subsystem1/Enable
  [CAN_id] -> Compare To Constant2/1
  [CAN_data] -> Subsystem1/1(In1)
  CAN Receive1/1 -> [CAN_id]  "CAN_ID"
  Subsystem1/1(Out1) -> Product/1
  Product/1 -> Selector3/1
  [isRunning] -> Product/2
  [isRunning] -> Product1/2
  Subsystem2/1(Out1) -> Product1/1
  Product1/1 -> Selector1/1
  Compare To Constant1/1 -> Subsystem2/Enable
  [CAN_data] -> Subsystem2/1(In1)
  [CAN_id] -> Compare To Constant1/1
  Selector3/1 -> [wheel_speed]  "wheel_speed [rpm]"
  Selector1/1 -> [meased_Iq]  "meased_Iq [A]"

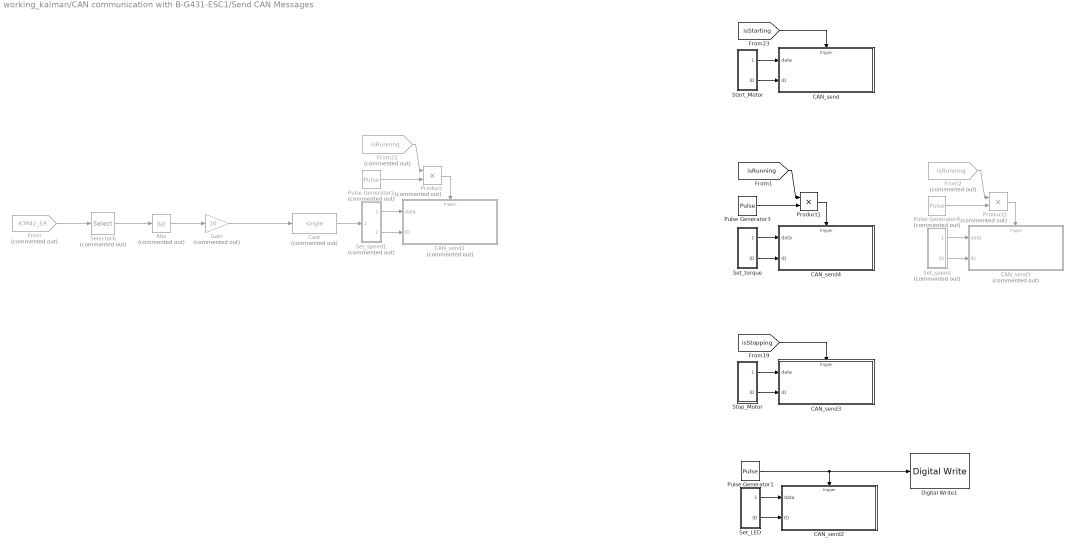
== system working_kalman/CAN communication with B-G431-ESC1/Send CAN Messages ==
  Abs : Abs  Commented=on  SaturateOnIntegerOverflow=off
  CAN_send : Subsystem
  CAN_send1 : Subsystem  Commented=on
  CAN_send2 : Subsystem
  CAN_send3 : Subsystem
  CAN_send4 : Subsystem
  CAN_send5 : Subsystem  Commented=on
  Cast : DataTypeConversion  Commented=on  OutDataTypeStr=single  SaturateOnIntegerOverflow=off  RndMeth=Floor
  Digital Write1 : mbedblockslib/Digital Write  Pin=LED1  Direction=output
      settings: LibrarySourceBlock=stmnucleorootlib/Common/Digital Write
  From : From  Commented=on  GotoTag=ICM42_EA  TagVisibility=global
  From2 : From  Commented=on  GotoTag=isRunning  TagVisibility=global
  From22 : From  Commented=on  GotoTag=isRunning  TagVisibility=global
  Gain : Gain  Commented=on  Gain=10
  Product : Product  Commented=on
  Product1 : Product
  Product2 : Product  Commented=on
  Pulse Generator1 : DiscretePulseGenerator  PulseType=Time based  Period=0.1  PulseWidth=50
  Pulse Generator2 : DiscretePulseGenerator  Commented=on  PulseType=Time based  Period=0.1  PulseWidth=50
  Pulse Generator3 : DiscretePulseGenerator  PulseType=Time based  Period=2*simulink_Ts  PulseWidth=50
  Pulse Generator4 : DiscretePulseGenerator  Commented=on  PulseType=Time based  Period=2*simulink_Ts  PulseWidth=50
  Selector6 : Selector  Commented=on  InputPortWidth=3  IndexOptions=Index vector (dialog)  Indices=[1]  OutputSizes=1
  Set_LED : Subsystem
  Set_speed : Subsystem  Commented=on
  Set_speed1 : Subsystem  Commented=on
  Set_torque : Subsystem
  Start_Motor : Subsystem
  Stop_Motor : Subsystem
  wires:
  Set_speed1/2(ID) -> CAN_send1/2(ID)
  Selector6/1 -> Abs/1
  Set_LED/1(data) -> CAN_send2/1(data)
  Stop_Motor/1(data) -> CAN_send3/1(data)
  Set_speed1/1(data) -> CAN_send1/1(data)
  [isStopping] -> CAN_send3/Trigger
  Pulse Generator1/1 -> Digital Write1/1, CAN_send2/Trigger
  Start_Motor/2(ID) -> CAN_send/2(ID)
  [isStarting] -> CAN_send/Trigger
  From22/1 -> Product/1
  Gain/1 -> Cast/1
  Start_Motor/1(data) -> CAN_send/1(data)
  Cast/1 -> Set_speed1/1(In1)
  Pulse Generator2/1 -> Product/2
  Abs/1 -> Gain/1
  Product/1 -> CAN_send1/Trigger
  Stop_Motor/2(ID) -> CAN_send3/2(ID)
  Set_LED/2(ID) -> CAN_send2/2(ID)
  From/1 -> Selector6/1
  Pulse Generator3/1 -> Product1/2
  [isRunning] -> Product1/1
  Set_torque/1(data) -> CAN_send4/1(data)
  Set_torque/2(ID) -> CAN_send4/2(ID)
  Product1/1 -> CAN_send4/Trigger
  Product2/1 -> CAN_send5/Trigger
  From2/1 -> Product2/1
  Pulse Generator4/1 -> Product2/2
  Set_speed/2(ID) -> CAN_send5/2(ID)
  Set_speed/1(data) -> CAN_send5/1(data)

== system working_kalman/ICM20948/Initialize MPU6050 ==
  Enable : EnablePort
  Accelerometer scale : mbedblockslib/I2C Controller Write  Commented=on  I2CModule=0  Mode=Master  SlaveAddress=hex2dec('68')  SlaveByteOrder=BigEndian  Direction=Transmitter  RegisterAddressMode=on  RegisterAddress=hex2dec('1C')  SlaveDataType=uint8  DataLength=2  NoAck=off  RepeatedStart=off  OutputStatus=on
      settings: LibrarySourceBlock=stmnucleorootlib/Common/I2C Controller Write
  Constant : Constant  Commented=on  Value=0b00000000
  Constant1 : Constant  Commented=on  Value=0b00001000
  Constant2 : Constant  Commented=on  Value=0b00010000
  Display1 : Display  Commented=on
  Display2 : Display  Commented=on
  Display5 : Display  Commented=on
  Gyroscope scale : mbedblockslib/I2C Controller Write  Commented=on  I2CModule=0  Mode=Master  SlaveAddress=hex2dec('68')  SlaveByteOrder=BigEndian  Direction=Transmitter  RegisterAddressMode=on  RegisterAddress=hex2dec('1B')  SlaveDataType=uint8  DataLength=2  NoAck=off  RepeatedStart=off  OutputStatus=on
      settings: LibrarySourceBlock=stmnucleorootlib/Common/I2C Controller Write
  Wake up : mbedblockslib/I2C Controller Write  Commented=on  I2CModule=0  Mode=Master  SlaveAddress=hex2dec('68')  SlaveByteOrder=BigEndian  Direction=Transmitter  RegisterAddressMode=on  RegisterAddress=hex2dec('6B')  SlaveDataType=uint8  DataLength=2  NoAck=off  RepeatedStart=off  OutputStatus=on
      settings: LibrarySourceBlock=stmnucleorootlib/Common/I2C Controller Write
  wires:
  Constant/1 -> Wake up/1
  Wake up/1 -> Display5/1
  Gyroscope scale/1 -> Display1/1
  Constant1/1 -> Gyroscope scale/1
  Constant2/1 -> Accelerometer scale/1
  Accelerometer scale/1 -> Display2/1

== system working_kalman/ICM20948/Read device address ==
  Enable : EnablePort
  Display1 : Display  Commented=on
  Display2 : Display
  Display3 : Display  Commented=on
  Scope1 : Scope  Commented=on
      settings: DataLoggingVariableName=ScopeData6
  Scope2 : Scope  Commented=on
      settings: DataLoggingVariableName=ScopeData7
  Scope3 : Scope
      settings: DataLoggingVariableName=ScopeData2
  WHO_AM_I_0x69 : mbedblockslib/I2C Controller Read  I2CModule=2  Mode=Master  SlaveAddress=hex2dec('69')  SlaveByteOrder=BigEndian  Direction=Receiver  RegisterAddressMode=on  RegisterAddress=hex2dec('0')  SlaveDataType=uint8  DataLength=1  NoAck=off  RepeatedStart=off  OutputStatus=on  SampleTime=0.1
      settings: LibrarySourceBlock=stmnucleorootlib/Common/I2C Controller Read
  acc_scale : mbedblockslib/I2C Controller Read  Commented=on  I2CModule=0  Mode=Master  SlaveAddress=hex2dec('68')  SlaveByteOrder=BigEndian  Direction=Receiver  RegisterAddressMode=on  RegisterAddress=hex2dec('1C')  SlaveDataType=int8  DataLength=1  NoAck=off  RepeatedStart=off  OutputStatus=on  SampleTime=20
      settings: LibrarySourceBlock=stmnucleorootlib/Common/I2C Controller Read
  gyr_scale : mbedblockslib/I2C Controller Read  Commented=on  I2CModule=0  Mode=Master  SlaveAddress=hex2dec('68')  SlaveByteOrder=BigEndian  Direction=Receiver  RegisterAddressMode=on  RegisterAddress=hex2dec('1B')  SlaveDataType=int8  DataLength=1  NoAck=off  RepeatedStart=off  OutputStatus=on  SampleTime=20
      settings: LibrarySourceBlock=stmnucleorootlib/Common/I2C Controller Read
  wires:
  WHO_AM_I_0x69/2 -> Display2/1
  WHO_AM_I_0x69/1 -> Scope3/1
  gyr_scale/1 -> Scope1/1
  gyr_scale/2 -> Display1/1
  acc_scale/1 -> Scope2/1
  acc_scale/2 -> Display3/1

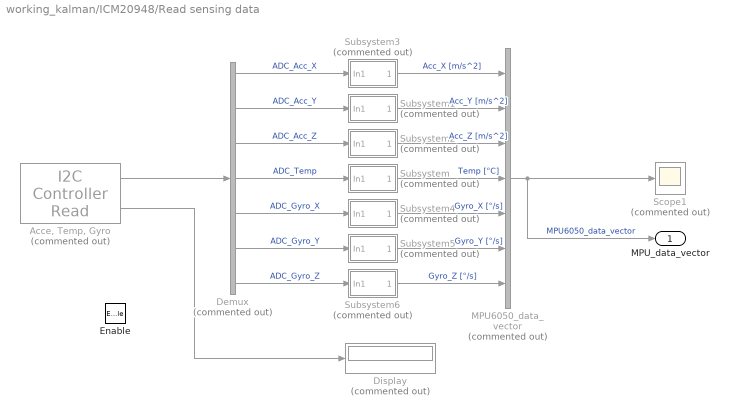
== system working_kalman/ICM20948/Read sensing data ==
  Enable : EnablePort
  "Acce, Temp, Gyro" : mbedblockslib/I2C Controller Read  Commented=on  I2CModule=0  Mode=Master  SlaveAddress=hex2dec('68')  SlaveByteOrder=BigEndian  Direction=Receiver  RegisterAddressMode=on  RegisterAddress=hex2dec('3B')  SlaveDataType=int16  DataLength=7  NoAck=off  RepeatedStart=off  OutputStatus=on  SampleTime=0.1
      settings: LibrarySourceBlock=stmnucleorootlib/Common/I2C Controller Read
  Demux : Demux  Commented=on  Outputs=7
  Display : Display  Commented=on
  MPU6050_data_vector : Mux  Commented=on  Inputs=7
  Scope1 : Scope  Commented=on
  Subsystem : Subsystem  Commented=on
  Subsystem1 : Subsystem  Commented=on
  Subsystem2 : Subsystem  Commented=on
  Subsystem3 : Subsystem  Commented=on
  Subsystem4 : Subsystem  Commented=on
  Subsystem5 : Subsystem  Commented=on
  Subsystem6 : Subsystem  Commented=on
  MPU_data_vector : Outport
  wires:
  "Acce, Temp, Gyro"/2 -> Display/1
  "Acce, Temp, Gyro"/1 -> Demux/1
  Demux/1 -> Subsystem3/1(In1)  "ADC_Acc_X"
  Demux/2 -> Subsystem1/1(In1)  "ADC_Acc_Y"
  Demux/3 -> Subsystem2/1(In1)  "ADC_Acc_Z"
  Demux/4 -> Subsystem/1(In1)  "ADC_Temp"
  Demux/5 -> Subsystem4/1(In1)  "ADC_Gyro_X"
  Demux/6 -> Subsystem5/1(In1)  "ADC_Gyro_Y"
  Demux/7 -> Subsystem6/1(In1)  "ADC_Gyro_Z"
  Subsystem6/1(Out1) -> MPU6050_data_vector/7  "Gyro_Z [°/s]"
  Subsystem5/1(Out1) -> MPU6050_data_vector/6  "Gyro_Y [°/s]"
  Subsystem4/1(Out1) -> MPU6050_data_vector/5  "Gyro_X [°/s]"
  Subsystem/1(Out1) -> MPU6050_data_vector/4  "Temp [°C]"
  Subsystem2/1(Out1) -> MPU6050_data_vector/3  "Acc_Z [m/s^2]"
  Subsystem1/1(Out1) -> MPU6050_data_vector/2  "Acc_Y [m/s^2]"
  Subsystem3/1(Out1) -> MPU6050_data_vector/1  "Acc_X [m/s^2]"
  MPU6050_data_vector/1 -> Scope1/1, MPU_data_vector/1  "MPU6050_data_vector"

== system working_kalman/ICM42688-P/Measurement ==
  Enable : EnablePort
  Demux : Demux  Outputs=7
  ICM42688-p_data_vector : Mux  Inputs=7
  Subsystem : Subsystem
  Subsystem1 : Subsystem
  Subsystem2 : Subsystem
  Subsystem3 : Subsystem
  Subsystem4 : Subsystem
  Subsystem5 : Subsystem
  Subsystem6 : Subsystem
  "Temp, Accel, Gyro" : mbedblockslib/SPI Register Read  Priority=1  SPIModule=0  Mode=Master  BusSpeed=uint32( 1000000 )  Pin=PA_4  FirstBitToTransfer=Most significant bit (MSB)  ClockMode=0  BlockFunction=Read  RegisterAddress=bitor(hex2dec('1D'), hex2dec('80'))  OutputDataType=int16  OutputDataLength=7  SampleTime=sensor_Ts  UseCustomSSPin=Explicit GPIO calls  ActiveLowSSPin=Active low
      settings: LibrarySourceBlock=stmnucleorootlib/Common/SPI Register Read
  ICM_data_vector : Outport
  wires:
  Demux/5 -> Subsystem4/1(In1)  "ADC_Gyro_X"
  Demux/7 -> Subsystem6/1(In1)  "ADC_Gyro_Z"
  Demux/6 -> Subsystem5/1(In1)  "ADC_Gyro_Y"
  Subsystem1/1(Out1) -> ICM42688-p_data_vector/2  "Acc_X [m/s^2]"
  Subsystem3/1(Out1) -> ICM42688-p_data_vector/4  "Acc_Z [m/s^2]"
  Subsystem5/1(Out1) -> ICM42688-p_data_vector/6  "Gyro_Y [°/s]"
  Demux/3 -> Subsystem2/1(In1)  "ADC_Acc_Y"
  Subsystem2/1(Out1) -> ICM42688-p_data_vector/3  "Acc_Y [m/s^2]"
  Subsystem6/1(Out1) -> ICM42688-p_data_vector/7  "Gyro_Z [°/s]"
  Demux/2 -> Subsystem1/1(In1)  "ADC_Acc_X"
  Subsystem4/1(Out1) -> ICM42688-p_data_vector/5  "Gyro_X [°/s]"
  Demux/1 -> Subsystem/1(In1)  "ADC_Temp"
  ICM42688-p_data_vector/1 -> ICM_data_vector/1  "ICM_data_vector"
  Subsystem/1(Out1) -> ICM42688-p_data_vector/1  "Temp [°C]"
  Demux/4 -> Subsystem3/1(In1)  "ADC_Acc_Z"
  "Temp, Accel, Gyro"/1 -> Demux/1  "16bit ADC"

== system working_kalman/ICM42688-P/Range and sensitivity ==
  Trigger : TriggerPort  VariantControl=(inherit)  PortDimensions=1
  "ACCEL_FS_SEL and ACCEL_ODR " : mbedblockslib/SPI Register Write  Priority=2  SPIModule=0  Mode=Master  BusSpeed=uint32( 1000000 )  Pin=PA_4  FirstBitToTransfer=Most significant bit (MSB)  ClockMode=0  BlockFunction=Write  RegisterAddress=hex2dec('50')  OutputDataType=int8  OutputDataLength=1  UseCustomSSPin=Explicit GPIO calls  ActiveLowSSPin=Active low
      settings: LibrarySourceBlock=stmnucleorootlib/Common/SPI Register Write
  "BEWARE the reserved bits (1000dps, 1kHz)" : Constant  Value=0b00100110  SampleTime=-1
  "BEWARE the reserved bits (8g, 1kHz)" : Constant  Value=0b00100110  SampleTime=-1
  "GYRO_FS_SEL and GYRO_ODR " : mbedblockslib/SPI Register Write  Priority=1  SPIModule=0  Mode=Master  BusSpeed=uint32( 1000000 )  Pin=PA_4  FirstBitToTransfer=Most significant bit (MSB)  ClockMode=0  BlockFunction=Write  RegisterAddress=hex2dec('4F')  OutputDataType=int8  OutputDataLength=1  UseCustomSSPin=Explicit GPIO calls  ActiveLowSSPin=Active low
      settings: LibrarySourceBlock=stmnucleorootlib/Common/SPI Register Write
  wires:
  "BEWARE the reserved bits (1000dps, 1kHz)"/1 -> "GYRO_FS_SEL and GYRO_ODR "/1
  "BEWARE the reserved bits (8g, 1kHz)"/1 -> "ACCEL_FS_SEL and ACCEL_ODR "/1

== system working_kalman/ICM42688-P/Waking up ==
  Trigger : TriggerPort  VariantControl=(inherit)  PortDimensions=1
  BEWARE the reserved bits : Constant  Value=0b00011111  SampleTime=-1
  SPI Register Write : mbedblockslib/SPI Register Write  SPIModule=0  Mode=Master  BusSpeed=uint32( 1000000 )  Pin=PA_4  FirstBitToTransfer=Most significant bit (MSB)  ClockMode=0  BlockFunction=Write  RegisterAddress=hex2dec('4E')  OutputDataType=int8  OutputDataLength=1  UseCustomSSPin=Explicit GPIO calls  ActiveLowSSPin=Active low
      settings: LibrarySourceBlock=stmnucleorootlib/Common/SPI Register Write
  wires:
  BEWARE the reserved bits/1 -> SPI Register Write/1

== system working_kalman/MPU6050/Initialize MPU6050 ==
  Enable : EnablePort
  Accelerometer scale : mbedblockslib/I2C Controller Write  I2CModule=0  Mode=Master  SlaveAddress=hex2dec('68')  SlaveByteOrder=BigEndian  Direction=Transmitter  RegisterAddressMode=on  RegisterAddress=hex2dec('1C')  SlaveDataType=uint8  DataLength=2  NoAck=off  RepeatedStart=off  OutputStatus=on
      settings: LibrarySourceBlock=stmnucleorootlib/Common/I2C Controller Write
  Constant : Constant  Value=0b00000000
  Constant1 : Constant  Value=0b00001000
  Constant2 : Constant  Value=0b00010000
  Gyroscope scale : mbedblockslib/I2C Controller Write  I2CModule=0  Mode=Master  SlaveAddress=hex2dec('68')  SlaveByteOrder=BigEndian  Direction=Transmitter  RegisterAddressMode=on  RegisterAddress=hex2dec('1B')  SlaveDataType=uint8  DataLength=2  NoAck=off  RepeatedStart=off  OutputStatus=on
      settings: LibrarySourceBlock=stmnucleorootlib/Common/I2C Controller Write
  Wake up : mbedblockslib/I2C Controller Write  I2CModule=0  Mode=Master  SlaveAddress=hex2dec('68')  SlaveByteOrder=BigEndian  Direction=Transmitter  RegisterAddressMode=on  RegisterAddress=hex2dec('6B')  SlaveDataType=uint8  DataLength=2  NoAck=off  RepeatedStart=off  OutputStatus=on
      settings: LibrarySourceBlock=stmnucleorootlib/Common/I2C Controller Write
  wires:
  Constant/1 -> Wake up/1
  Constant1/1 -> Gyroscope scale/1
  Constant2/1 -> Accelerometer scale/1

== system working_kalman/MPU6050/Read device address ==
  Enable : EnablePort
  WHO_AM_I : mbedblockslib/I2C Controller Read  I2CModule=0  Mode=Master  SlaveAddress=hex2dec('68')  SlaveByteOrder=BigEndian  Direction=Receiver  RegisterAddressMode=on  RegisterAddress=hex2dec('75')  SlaveDataType=int8  DataLength=1  NoAck=off  RepeatedStart=off  OutputStatus=on  SampleTime=20
      settings: LibrarySourceBlock=stmnucleorootlib/Common/I2C Controller Read
  acc_scale : mbedblockslib/I2C Controller Read  I2CModule=0  Mode=Master  SlaveAddress=hex2dec('68')  SlaveByteOrder=BigEndian  Direction=Receiver  RegisterAddressMode=on  RegisterAddress=hex2dec('1C')  SlaveDataType=int8  DataLength=1  NoAck=off  RepeatedStart=off  OutputStatus=on  SampleTime=20
      settings: LibrarySourceBlock=stmnucleorootlib/Common/I2C Controller Read
  gyr_scale : mbedblockslib/I2C Controller Read  I2CModule=0  Mode=Master  SlaveAddress=hex2dec('68')  SlaveByteOrder=BigEndian  Direction=Receiver  RegisterAddressMode=on  RegisterAddress=hex2dec('1B')  SlaveDataType=int8  DataLength=1  NoAck=off  RepeatedStart=off  OutputStatus=on  SampleTime=20
      settings: LibrarySourceBlock=stmnucleorootlib/Common/I2C Controller Read

== system working_kalman/MPU6050/Read sensing data ==
  Enable : EnablePort
  "Acce, Temp, Gyro" : mbedblockslib/I2C Controller Read  I2CModule=0  Mode=Master  SlaveAddress=hex2dec('68')  SlaveByteOrder=BigEndian  Direction=Receiver  RegisterAddressMode=on  RegisterAddress=hex2dec('3B')  SlaveDataType=int16  DataLength=7  NoAck=off  RepeatedStart=off  OutputStatus=on  SampleTime=sensor_Ts
      settings: LibrarySourceBlock=stmnucleorootlib/Common/I2C Controller Read
  Demux : Demux  Outputs=7
  MPU6050_data_vector : Mux  Inputs=7
  Subsystem : Subsystem
  Subsystem1 : Subsystem
  Subsystem2 : Subsystem
  Subsystem3 : Subsystem
  Subsystem4 : Subsystem
  Subsystem5 : Subsystem
  Subsystem6 : Subsystem
  MPU_data_vector : Outport
  wires:
  "Acce, Temp, Gyro"/1 -> Demux/1
  Demux/1 -> Subsystem3/1(In1)  "ADC_Acc_X"
  Demux/2 -> Subsystem1/1(In1)  "ADC_Acc_Y"
  Demux/3 -> Subsystem2/1(In1)  "ADC_Acc_Z"
  Demux/4 -> Subsystem/1(In1)  "ADC_Temp"
  Demux/5 -> Subsystem4/1(In1)  "ADC_Gyro_X"
  Demux/6 -> Subsystem5/1(In1)  "ADC_Gyro_Y"
  Demux/7 -> Subsystem6/1(In1)  "ADC_Gyro_Z"
  Subsystem6/1(Out1) -> MPU6050_data_vector/7  "Gyro_Z [°/s]"
  Subsystem5/1(Out1) -> MPU6050_data_vector/6  "Gyro_Y [°/s]"
  Subsystem4/1(Out1) -> MPU6050_data_vector/5  "Gyro_X [°/s]"
  Subsystem/1(Out1) -> MPU6050_data_vector/4  "Temp [°C]"
  Subsystem2/1(Out1) -> MPU6050_data_vector/3  "Acc_Z [m/s^2]"
  Subsystem1/1(Out1) -> MPU6050_data_vector/2  "Acc_Y [m/s^2]"
  Subsystem3/1(Out1) -> MPU6050_data_vector/1  "Acc_X [m/s^2]"
  MPU6050_data_vector/1 -> MPU_data_vector/1  "MPU6050_data_vector"

== system working_kalman/Regulation for Edge Balancing/Friction2 ==
  rad/s : Inport
  Gain : Gain  Gain=300
  Gain1 : Gain  Gain=friction_offset
  Gain2 : Gain  Gain=friction_slope
  Gain4 : Gain  Gain=1/(2*pi*60)
  Sum : Sum  Inputs=|++
  Tanh : Trigonometry  Operator=tanh
  friction : Outport
  wires:
  rad/s/1 -> Gain4/1
  Gain4/1 -> Gain2/1, Gain/1  "rpm"
  Gain1/1 -> Sum/1
  Tanh/1 -> Gain1/1
  Gain2/1 -> Sum/2
  Gain/1 -> Tanh/1
  Sum/1 -> friction/1

== system working_kalman/Regulation for Edge Balancing/Friction3 ==
  rad/s : Inport
  Gain : Gain  Gain=300
  Gain1 : Gain  Gain=friction_offset
  Gain2 : Gain  Gain=friction_slope
  Gain4 : Gain  Gain=1/(2*pi*60)
  Sum : Sum  Inputs=|++
  Tanh : Trigonometry  Operator=tanh
  friction : Outport
  wires:
  rad/s/1 -> Gain4/1
  Gain4/1 -> Gain2/1, Gain/1  "rpm"
  Gain1/1 -> Sum/1
  Tanh/1 -> Gain1/1
  Gain2/1 -> Sum/2
  Gain/1 -> Tanh/1
  Sum/1 -> friction/1

== system working_kalman/Sensor Calibration and Averaging/Subsystem1 ==
  data : Inport
  Enable : EnablePort
  2-D Mean3 : visionstatistics/2-D Mean  run=on  reset_popup=Rising edge  directionMode=Each row  dimension=1  treatSBRowAsCol=on  outputLastDataTypeStr=Inherit: Same as accumulator  accumMode=Binary point scaling  accumWordLength=32  accumFracLength=0  accumLastDataTypeStr=fixdt([],32,0)  roiEnable=off  roiType=Rectangles  roiPortion=Entire ROI  roiOutput=Individual statistics for each ROI  roiFlag=off  roundingMode=Floor  overflowMode=off  accumDataTypeStr=fixdt([],32,0)  outputDataTypeStr=Inherit: Same as accumulator  outputMin=[]  outputMax=[]
  Cast To Boolean : DataTypeConversion  OutDataTypeStr=boolean  SaturateOnIntegerOverflow=off  RndMeth=Floor
  Sum of Elements : Sum  Inputs=+
  data_mean : Outport
  wires:
  2-D Mean3/1 -> data_mean/1
  data/1 -> 2-D Mean3/1, Sum of Elements/1
  Sum of Elements/1 -> Cast To Boolean/1
  Cast To Boolean/1 -> 2-D Mean3/2
